simulink model "CarSimModel"  (Simulink 6.3)
settings: Solver=ode45  StartTime=0  StopTime=3  FixedStep=.01  RelTol=1e-3
PostLoadFcn:
  | CarSim(gcs)
InitFcn:
  | load('C:\Documents and Settings\jminor\Desktop\ACSYS\CarSim\CarSim.4\Data\TempModelParameters.mat')
undefined symbols (not defined in the file or in its folder): Bm, c, Jm, k, Kamp, Kb, Km, Ks, La, M, r, Ra
libraries: simulink_extras x1
CloseFcn:
  | CarSim('CloseFcn', [], [], [], [])
settings Model: LastModifiedBy=jminor  BufferReuse=off  StrictBusMsg=None
settings DataIOCC: SaveOutput=off  SaveTime=off  SignalLoggingName=sigsOut
settings OptimizationCC: OptimizeBlockIOStorage=off  BufferReuse=off  ExpressionFolding=off  LocalBlockOutputs=off
settings DebuggingCC: SolverPrmCheckMsg=none
settings HardwareCC: TargetUnknown=on
settings CodeAppCC: IgnoreCustomStorageClasses=off

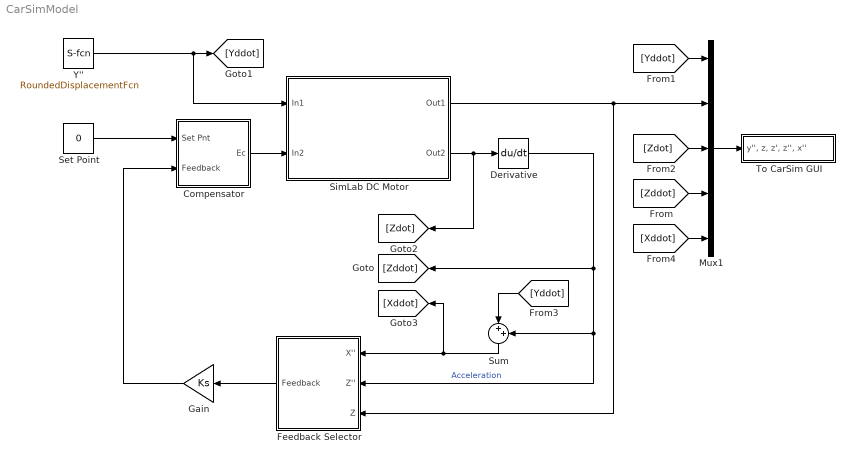
== system CarSimModel ==
  Compensator : Subsystem
  Derivative : Derivative
  Feedback Selector : Subsystem  Orientation=left
  Gain : Gain  Orientation=left  Gain=Ks  SaturateOnIntegerOverflow=on
  Mux1 : Mux  Inputs=5
  Set Point : Constant  Value=0
  SimLab DC Motor : Subsystem
      settings: NameChangeFcn=CarSim('BlockNameChange', gcb, 'PlantBlock', [], [])
      mask Display:
      | port_label('input', 1, 'Base Accel')
      | port_label('input', 2, 'Voltage')
      | port_label('output', 1, 'Position')
      | port_label('output', 2, 'Speed')
  Sum : Sum  Orientation=down  Inputs=|++  SaturateOnIntegerOverflow=on
  To CarSim GUI : Subsystem
      settings: NameChangeFcn=CarSim('BlockNameChange', gcb, 'CarSimBlock', [], [])
  Y'' : S-Function  FunctionName=RoundedDisplacementFcn  Parameters=X, gw, Output, SampleTime  mask(Rounded Displacement (RD)){X=-3, gw=62.8319, Output=Acceleration, SampleTime=0}
      mask prompts: X "Amplitude:"; gw "Gamma*Omega:"; Output "Block Output:"; SampleTime "Sample Time"
      mask help: Output either the position, velocity or acceleration of the Rounded Displacement function.
      mask init:
      | t = [0:0.01:1];
      | y = 1-(1+t.*8).*exp(-t.*8);
      settings: NameChangeFcn=CarSim('BlockNameChange', gcb, 'DistBlock', [], [])
      mask Help:
      | Generate RD(t), RD'(t), or RD''(t).
      | 
      | 
      | Description:
      | RD(t) = A*(1-(1+gwt)e^(-gwt)), where A is the amplitude, g (gamma) is the intensity factor, w (omega) is the circular frequency.
      | 
      | 
      | Amplitude:
      | The amplitude of the pulse, a real number.
      | 
      | gw:
      | The intensity factor multiplied by the frequency (gamma*omega), where T = (2*pi)/gw.
      | 
      | Output:
      | Select whether to output the RD, or its first or second derivative (ie. position, velocity, or acceleration).
      mask StyleString: edit,edit,popup(Position|Velocity|Acceleration),edit
      mask Display: plot(t,y)
  wires:
  Mux1/1 -> To CarSim GUI/1("y'', z, z', z'', x''")
  SimLab DC Motor/1(Out1) -> Mux1/2, Feedback Selector/3(Z)
  Compensator/1(Ec) -> SimLab DC Motor/2(In2)
  [Zddot] -> Mux1/4
  [Yddot] -> Mux1/1
  [Zdot] -> Mux1/3
  SimLab DC Motor/2(Out2) -> Derivative/1, [Zdot]
  Derivative/1 -> [Zddot], Feedback Selector/2(Z''), Sum/2  "Acceleration"
  Set Point/1 -> Compensator/1(Set Pnt)
  [Yddot] -> Sum/1
  [Xddot] -> Mux1/5
  Y''/1 -> [Yddot], SimLab DC Motor/1(In1)
  Feedback Selector/1(Feedback) -> Gain/1
  Sum/1 -> Feedback Selector/1(X''), [Xddot]
  Gain/1 -> Compensator/2(Feedback)

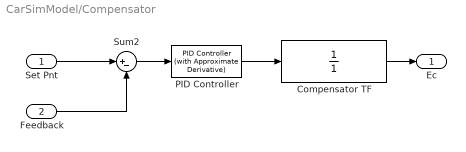
== system CarSimModel/Compensator ==
  Set Pnt : Inport
  Feedback : Inport  Port=2
  Compensator TF : TransferFcn  Denominator=[1]
  PID Controller : simulink_extras/Additional Linear/PID Controller (with Approximate Derivative)  P=275  I=0  D=12  N=100
  Sum2 : Sum  Inputs=|+-  SaturateOnIntegerOverflow=on
  Ec : Outport
  wires:
  Set Pnt/1 -> Sum2/1
  Sum2/1 -> PID Controller/1
  PID Controller/1 -> Compensator TF/1
  Feedback/1 -> Sum2/2
  Compensator TF/1 -> Ec/1

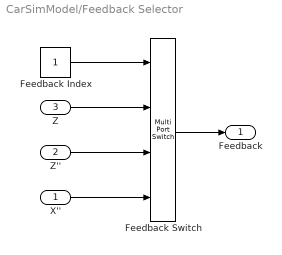
== system CarSimModel/Feedback Selector ==
  X'' : Inport
  Z'' : Inport  Port=2
  Z : Inport  Port=3
  Feedback Index : Constant
  Feedback Switch : MultiPortSwitch  Inputs=3  SaturateOnIntegerOverflow=on
  Feedback : Outport
  wires:
  Feedback Switch/1 -> Feedback/1
  Z''/1 -> Feedback Switch/3
  Feedback Index/1 -> Feedback Switch/1
  Z/1 -> Feedback Switch/2
  X''/1 -> Feedback Switch/4

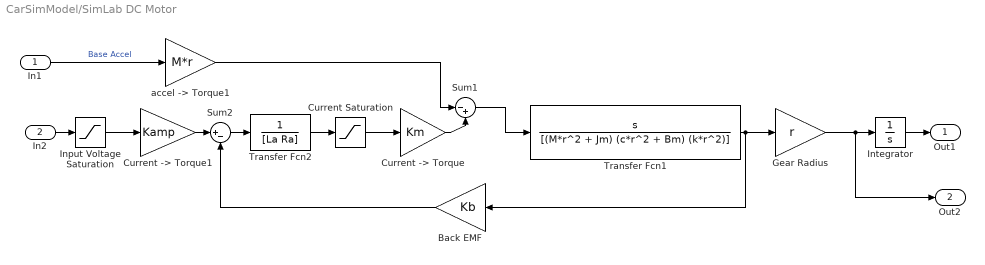
== system CarSimModel/SimLab DC Motor ==
  In1 : Inport
  In2 : Inport  Port=2
  Back EMF : Gain  Orientation=left  Gain=Kb  SaturateOnIntegerOverflow=on
  Current Saturation : Saturate  UpperLimit=+4  LowerLimit=-4
  "Current -> Torque" : Gain  Gain=Km  SaturateOnIntegerOverflow=on
  "Current -> Torque1" : Gain  Gain=Kamp  SaturateOnIntegerOverflow=on
  Gear Radius : Gain  Gain=r  SaturateOnIntegerOverflow=on
  Input Voltage Saturation : Saturate  UpperLimit=+10  LowerLimit=-10
  Integrator : Integrator
  Sum1 : Sum  Inputs=|-+  SaturateOnIntegerOverflow=on
  Sum2 : Sum  Inputs=|+-  SaturateOnIntegerOverflow=on
  Transfer Fcn1 : TransferFcn  Numerator=[1 0]  Denominator=[(M*r^2 + Jm) (c*r^2 + Bm) (k*r^2)]
  Transfer Fcn2 : TransferFcn  Denominator=[La Ra]
  "accel -> Torque1" : Gain  Gain=M*r  SaturateOnIntegerOverflow=on
  Out1 : Outport
  Out2 : Outport  Port=2
  wires:
  "accel -> Torque1"/1 -> Sum1/1
  Gear Radius/1 -> Out2/1, Integrator/1
  Integrator/1 -> Out1/1
  Sum1/1 -> Transfer Fcn1/1
  Transfer Fcn1/1 -> Gear Radius/1, Back EMF/1
  In2/1 -> Input Voltage Saturation/1
  In1/1 -> "accel -> Torque1"/1  "Base Accel"
  Transfer Fcn2/1 -> Current Saturation/1
  Sum2/1 -> Transfer Fcn2/1
  Back EMF/1 -> Sum2/2
  "Current -> Torque1"/1 -> Sum2/1
  Current Saturation/1 -> "Current -> Torque"/1
  Input Voltage Saturation/1 -> "Current -> Torque1"/1
  "Current -> Torque"/1 -> Sum1/2

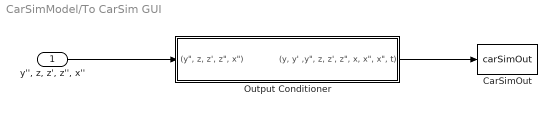
== system CarSimModel/To CarSim GUI ==
  "y'', z, z', z'', x''" : Inport
  CarSimOut : ToWorkspace  VariableName=carSimOut  SampleTime=-1  SaveFormat=Array
      settings: StopFcn=CarSim('StoreSimResults',2, guidata(2),carSimOut); clear carSimOut;  NameChangeFcn=CarSim('BlockNameChange', gcb, 'CarSimOut', [], [])
  Output Conditioner : Subsystem
      settings: NameChangeFcn=CarSim('BlockNameChange', gcb, 'OutputConditioner', [], [])
  wires:
  "y'', z, z', z'', x''"/1 -> Output Conditioner/1("(y\", z, z', z\", x\")")
  Output Conditioner/1("(y, y' ,y\", z, z', z\", x, x\", x\", t)") -> CarSimOut/1

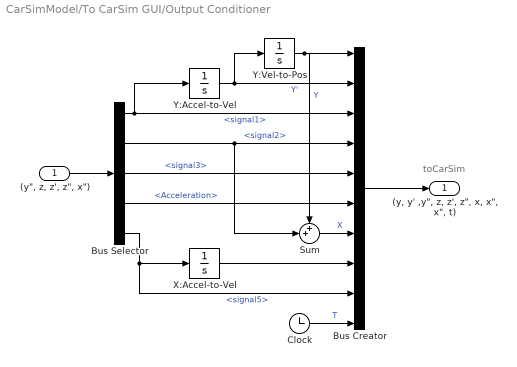
== system CarSimModel/To CarSim GUI/Output Conditioner ==
  note: toCarSim
  "(y\", z, z', z\", x\")" : Inport
  Bus Creator : BusCreator  Inputs=10
  Bus Selector : BusSelector  OutputSignals=signal1,signal2,signal3,Acceleration,signal5
  Clock : Clock
      settings: Decimation=10
  Sum : Sum  Inputs=++|
  X:Accel-to-Vel : Integrator
  Y:Accel-to-Vel : Integrator
  Y:Vel-to-Pos : Integrator
  "(y, y' ,y\", z, z', z\", x, x\", x\", t)" : Outport  PortDimensions=10
  wires:
  "(y\", z, z', z\", x\")"/1 -> Bus Selector/1
  Bus Selector/1 -> Y:Accel-to-Vel/1, Bus Creator/3  "<signal1>"
  Y:Accel-to-Vel/1 -> Y:Vel-to-Pos/1, Bus Creator/2  "Y'"
  Bus Creator/1 -> "(y, y' ,y\", z, z', z\", x, x\", x\", t)"/1
  Y:Vel-to-Pos/1 -> Bus Creator/1, Sum/1  "Y"
  Bus Selector/2 -> Bus Creator/4, Sum/2  "<signal2>"
  Bus Selector/5 -> Bus Creator/9, X:Accel-to-Vel/1  "<signal5>"
  Bus Selector/4 -> Bus Creator/6  "<Acceleration>"
  Bus Selector/3 -> Bus Creator/5  "<signal3>"
  Clock/1 -> Bus Creator/10  "T"
  Sum/1 -> Bus Creator/7  "X"
  X:Accel-to-Vel/1 -> Bus Creator/8
